simulink model "SimModel"  (R2024b)
settings: Solver=VariableStepAuto  StartTime=0.0  StopTime=10.0  RelTol=1e-3
settings Model: Creator=xinxing  LastModifiedBy=xinxing

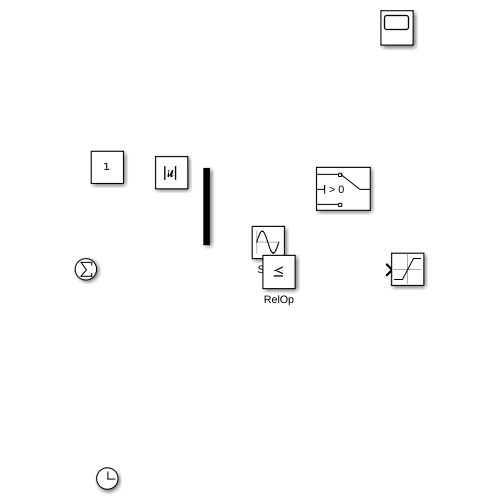
[thumbnail: Simulink's stored preview of the top-level diagram]
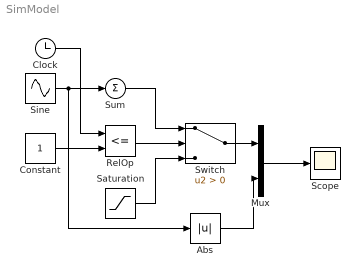
== system SimModel ==
  Abs : Abs  SaturateOnIntegerOverflow=off
  Clock : Clock
  Constant : Constant
  Mux : Mux  Inputs=2
  RelOp : RelationalOperator  Operator=<=  OutDataTypeStr=boolean  RndMeth=Simplest  InputSameDT=off
  Saturation : Saturate
  Scope : Scope
  Sine : Sin  SampleTime=0
  Sum : Sum  Inputs=+
  Switch : Switch  Criteria=u2 > Threshold  SaturateOnIntegerOverflow=off  InputSameDT=off
  wires:
  Mux/1 -> Scope/1
  Abs/1 -> Mux/2
  Switch/1 -> Mux/1
  RelOp/1 -> Switch/2
  Saturation/1 -> Switch/3
  Sum/1 -> Switch/1
  Constant/1 -> RelOp/2
  Sine/1 -> Sum/1, Abs/1
  Clock/1 -> RelOp/1
